simulink model "boggieDynamics_2021"  (Simulink 10.3)
settings: Solver=VariableStepAuto  StartTime=0.0  StopTime=10.0  RelTol=1e-3
undefined symbols (not defined in the file or in its folder): cg_suelo, g, m, x_guid12, x_guid34, x_lev12, x_lev34, y_lev13, y_lev24, z_guid, z_lev, z_lim
libraries: shared6dof x1
settings Model: Creator=aceao  LastModifiedBy=aceao
settings SolverCC: AlgebraicLoopSolver=Auto
settings DataIOCC: SaveFormat=Dataset  SignalLoggingSaveFormat=Dataset  ReturnWorkspaceOutputs=on
settings OptimizationCC: BlockReduction=off  BooleanDataType=off  ExpressionDepthLimit=128  LifeSpan=auto
settings DebuggingCC: SaveWithParameterizedLinksMsg=none  UnderspecifiedInitializationDetection=Simplified  SignalResolutionControl=TryResolveAllWithWarning  FcnCallInpInsideContextMsg=error  UnconnectedInputMsg=none  UnconnectedOutputMsg=none  UnconnectedLineMsg=none  StateNameClashWarn=none  SFUnexpectedBacktrackingDiag=error  SFNoUnconditionalDefaultTransitionDiag=error  SFExecutionAtInitializationDiag=warning  SFMachineParentedDataDiag=error  ArithmeticOperatorsInVariantConditions=error
settings HardwareCC: ProdBitPerPointer=64  ProdBitPerSizeT=64  ProdBitPerPtrDiffT=64  ProdLargestAtomicFloat=Float  ProdIntDivRoundTo=Zero  ProdEndianess=LittleEndian  ProdWordSize=64  ProdHWDeviceType=Intel->x86-64 (Windows64)  TargetUnknown=on
settings ModelReferenceCC: EnableRefExpFcnMdlSchedulingChecks=off
settings SFSimCC: SimUseLocalCustomCode=on  CustomCodeUndefinedFunction=FilterOut
settings RTWCC: RTWUseLocalCustomCode=on  DLArmComputeVersion=20.02.1
settings CodeAppCC: StateflowObjectComments=off
settings GRTTargetCC: TargetLangStandard=C99 (ISO)  CombineOutputUpdateFcns=on  GRTInterface=off
settings ConfigComp: CovMetricSettings=dwe  CovSaveCumulativeToWorkspaceVar=off  CovSaveSingleToWorkspaceVar=off  CovExternalEMLEnable=on

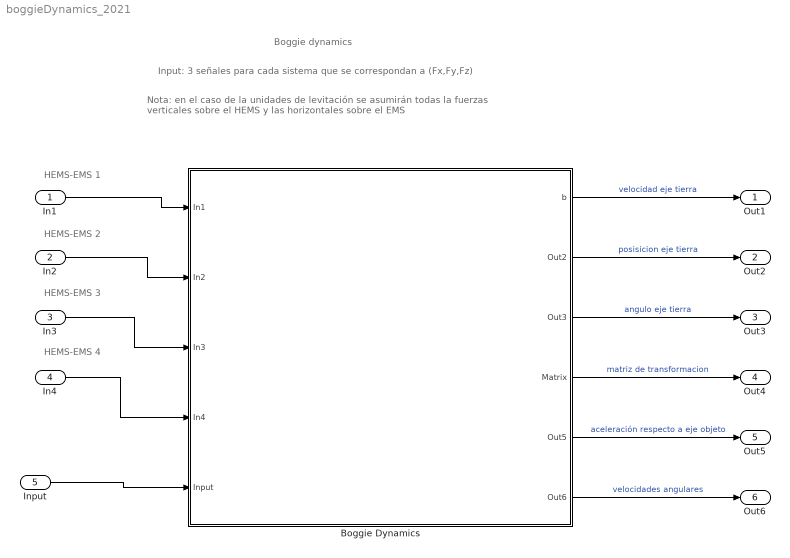
== system boggieDynamics_2021 ==
  note: Input: 3 señales para cada sistema que se correspondan a (Fx,Fy,Fz)
  note: Boggie dynamics
  note: HEMS-EMS 3
  note: HEMS-EMS 1
  note: HEMS-EMS 4
  note: HEMS-EMS 2
  note: Nota: en el caso de la unidades de levitación se asumirán todas la fuerzas
      | verticales sobre el HEMS y las horizontales sobre el EMS
  In1 : Inport
  In2 : Inport  Port=2
  In3 : Inport  Port=3
  In4 : Inport  Port=4
  Input : Inport  Port=5
  Boggie Dynamics : Subsystem
      mask Display: image('C:\UPV\Hyperloop\Levitacion\ejes.png'); % Use "Edit Image" on toolstrip to change.
  Out1 : Outport
  Out2 : Outport  Port=2
  Out3 : Outport  Port=3
  Out4 : Outport  Port=4
  Out5 : Outport  Port=5
  Out6 : Outport  Port=6
  wires:
  Boggie Dynamics/2(Out2) -> Out2/1  "posisicion eje tierra"
  Boggie Dynamics/3(Out3) -> Out3/1  "angulo eje tierra"
  Boggie Dynamics/1(b) -> Out1/1  "velocidad eje tierra"
  In1/1 -> Boggie Dynamics/1(In1)
  In2/1 -> Boggie Dynamics/2(In2)
  In3/1 -> Boggie Dynamics/3(In3)
  In4/1 -> Boggie Dynamics/4(In4)
  Boggie Dynamics/6(Out6) -> Out6/1  "velocidades angulares"
  Boggie Dynamics/5(Out5) -> Out5/1  "aceleración respecto a eje objeto"
  Boggie Dynamics/4(Matrix) -> Out4/1  "matriz de transformacion"
  Input/1 -> Boggie Dynamics/5(Input)

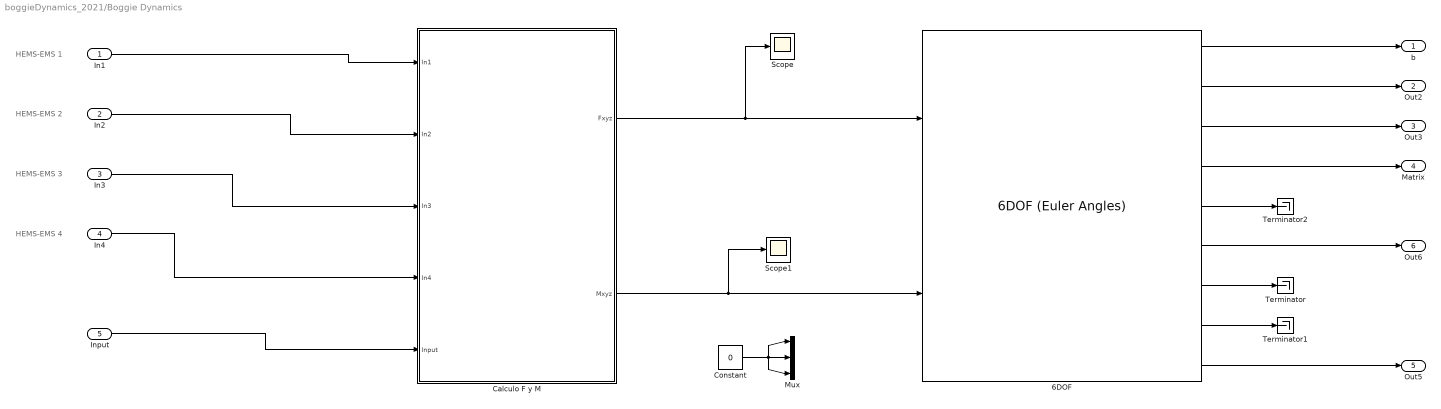
== system boggieDynamics_2021/Boggie Dynamics ==
  note: HEMS-EMS 1
  note: HEMS-EMS 2
  note: HEMS-EMS 3
  note: HEMS-EMS 4
  In1 : Inport
  In2 : Inport  Port=2
  In3 : Inport  Port=3
  In4 : Inport  Port=4
  Input : Inport  Port=5
  "6DOF " : shared6dof/6DOF (Euler Angles)  units=Metric (MKS)  mtype=Fixed  rep=Euler Angles  xme_0=[0 0.001 cg_suelo]  Vm_0=[0 0 0]  eul_0=[0 0 0]  pm_0=[0 0 0]  mass_0=m  mass_e=0.5  mass_f=2.0  inertia=I  inertia_e=eye(3)  inertia_f=2*eye(3)  k_quat=1.0  vre_flag=on  abi_flag=on  aMode=0  xme_statename=''  Vm_statename=''  eul_statename=''  quat_statename=''  pm_statename=''  mass_statename=''
  Calculo F y M : Subsystem
  Constant : Constant  Value=0
  Mux : Mux  Inputs=3
  Scope : Scope
  Scope1 : Scope
  Terminator : Terminator
  Terminator1 : Terminator
  Terminator2 : Terminator
  b : Outport
  Out2 : Outport  Port=2
  Out3 : Outport  Port=3
  Matrix : Outport  Port=4
  Out5 : Outport  Port=5
  Out6 : Outport  Port=6
  wires:
  "6DOF "/1 -> b/1
  "6DOF "/2 -> Out2/1
  "6DOF "/3 -> Out3/1
  In1/1 -> Calculo F y M/1(In1)
  In2/1 -> Calculo F y M/2(In2)
  In3/1 -> Calculo F y M/3(In3)
  In4/1 -> Calculo F y M/4(In4)
  "6DOF "/6 -> Out6/1
  "6DOF "/8 -> Terminator1/1
  "6DOF "/7 -> Terminator/1
  Calculo F y M/1(Fxyz) -> Scope/1, "6DOF "/1
  "6DOF "/4 -> Matrix/1
  "6DOF "/9 -> Out5/1
  "6DOF "/5 -> Terminator2/1
  Constant/1 -> Mux/3, Mux/1, Mux/2
  Input/1 -> Calculo F y M/5(Input)
  Calculo F y M/2(Mxyz) -> Scope1/1, "6DOF "/2

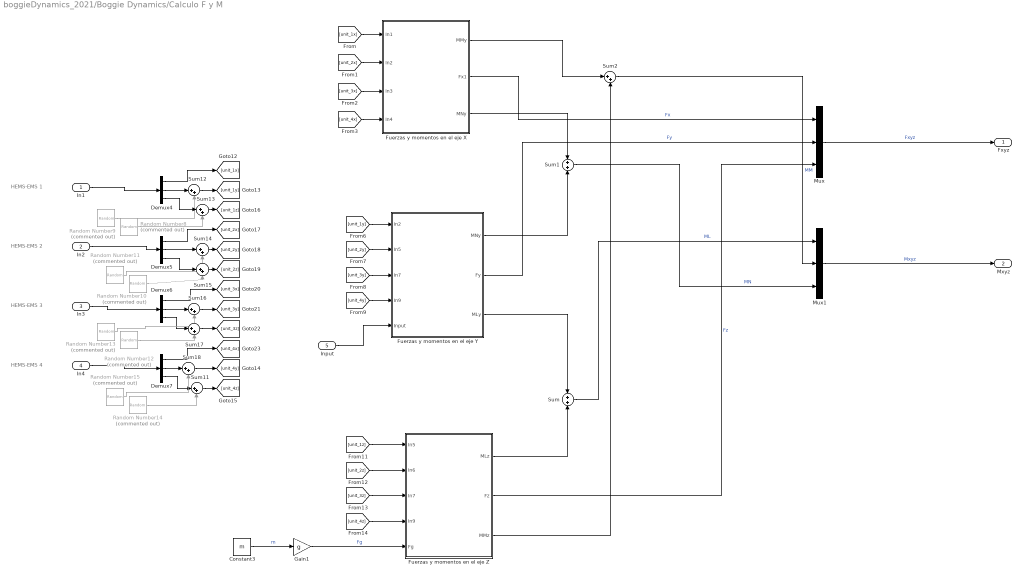
== system boggieDynamics_2021/Boggie Dynamics/Calculo F y M ==
  note: HEMS-EMS 3
  note: HEMS-EMS 1
  note: HEMS-EMS 4
  note: HEMS-EMS 2
  In1 : Inport
  In2 : Inport  Port=2
  In3 : Inport  Port=3
  In4 : Inport  Port=4
  Input : Inport  Port=5
  Constant3 : Constant  Value=m
  Demux{4..7} (4 alike) : Demux  Outputs=3
  Fuerzas y momentos en el eje X : Subsystem
  Fuerzas y momentos en el eje Y : Subsystem
  Fuerzas y momentos en el eje Z : Subsystem
  Gain1 : Gain  Gain=g
  Mux : Mux  Inputs=3
  Mux1 : Mux  Inputs=3
  Random Number10 : RandomNumber  Commented=on  Variance=20  Seed=3  SampleTime=0.1
  Random Number11 : RandomNumber  Commented=on  Variance=20  Seed=2  SampleTime=0.1
  Random Number12 : RandomNumber  Commented=on  Variance=20  Seed=5  SampleTime=0.1
  Random Number13 : RandomNumber  Commented=on  Variance=20  Seed=4  SampleTime=0.1
  Random Number14 : RandomNumber  Commented=on  Variance=20  Seed=7  SampleTime=0.1
  Random Number15 : RandomNumber  Commented=on  Variance=20  Seed=6  SampleTime=0.1
  Random Number8 : RandomNumber  Commented=on  Variance=20  Seed=1  SampleTime=0.1
  Random Number9 : RandomNumber  Commented=on  Variance=20  SampleTime=0.1
  Sum : Sum
  Sum1 : Sum
  Sum{2,11..18} (9 alike) : Sum  Inputs=|++
  Fxyz : Outport
  Mxyz : Outport  Port=2
  wires:
  Constant3/1 -> Gain1/1  "m"
  Sum2/1 -> Mux1/2  "MM"
  Mux/1 -> Fxyz/1  "Fxyz"
  Mux1/1 -> Mxyz/1  "Mxyz"
  Sum1/1 -> Mux1/3  "MN"
  Sum/1 -> Mux1/1  "ML"
  Fuerzas y momentos en el eje Y/2(Fy) -> Mux/2  "Fy"
  Fuerzas y momentos en el eje Y/1(MNy) -> Sum1/2
  Gain1/1 -> Fuerzas y momentos en el eje Z/5(Fg)  "Fg"
  Fuerzas y momentos en el eje Z/2(Fz) -> Mux/3  "Fz"
  Fuerzas y momentos en el eje Z/1(MLz) -> Sum/2
  [unit_4y] -> Fuerzas y momentos en el eje Y/4(In9)
  [unit_1y] -> Fuerzas y momentos en el eje Y/1(In2)
  [unit_2y] -> Fuerzas y momentos en el eje Y/2(In5)
  [unit_3y] -> Fuerzas y momentos en el eje Y/3(In7)
  [unit_1z] -> Fuerzas y momentos en el eje Z/1(In5)
  [unit_3z] -> Fuerzas y momentos en el eje Z/3(In7)
  [unit_2z] -> Fuerzas y momentos en el eje Z/2(In6)
  [unit_4z] -> Fuerzas y momentos en el eje Z/4(In9)
  Fuerzas y momentos en el eje Z/3(MMz) -> Sum2/2
  Fuerzas y momentos en el eje Y/3(MLy) -> Sum/1
  [unit_2x] -> Fuerzas y momentos en el eje X/2(In2)
  [unit_1x] -> Fuerzas y momentos en el eje X/1(In1)
  [unit_3x] -> Fuerzas y momentos en el eje X/3(In3)
  [unit_4x] -> Fuerzas y momentos en el eje X/4(In4)
  Fuerzas y momentos en el eje X/3(MNy) -> Sum1/1
  Fuerzas y momentos en el eje X/2(Fx1) -> Mux/1  "Fx"
  Fuerzas y momentos en el eje X/1(MMy) -> Sum2/1
  Input/1 -> Fuerzas y momentos en el eje Y/5(Input)
  Random Number9/1 -> Sum12/2
  Sum17/1 -> [unit_3z]
  Sum18/1 -> [unit_4y]
  Sum15/1 -> [unit_2z]
  Sum14/1 -> [unit_2y]
  Sum11/1 -> [unit_4z]
  Sum16/1 -> [unit_3y]
  Demux5/1 -> [unit_2x]
  Sum13/1 -> [unit_1z]
  Demux4/1 -> [unit_1x]
  Demux7/2 -> Sum18/1
  In1/1 -> Demux4/1
  Demux5/3 -> Sum15/1
  Demux6/2 -> Sum16/1
  Demux7/1 -> [unit_4x]
  Demux5/2 -> Sum14/1
  In4/1 -> Demux7/1
  In2/1 -> Demux5/1
  Sum12/1 -> [unit_1y]
  Demux7/3 -> Sum11/1
  Demux6/3 -> Sum17/1
  Random Number11/1 -> Sum14/2
  Random Number8/1 -> Sum13/2
  Demux4/2 -> Sum12/1
  Random Number15/1 -> Sum18/2
  Demux4/3 -> Sum13/1
  Demux6/1 -> [unit_3x]
  Random Number13/1 -> Sum16/2
  Random Number14/1 -> Sum11/2
  In3/1 -> Demux6/1
  Random Number10/1 -> Sum15/2
  Random Number12/1 -> Sum17/2

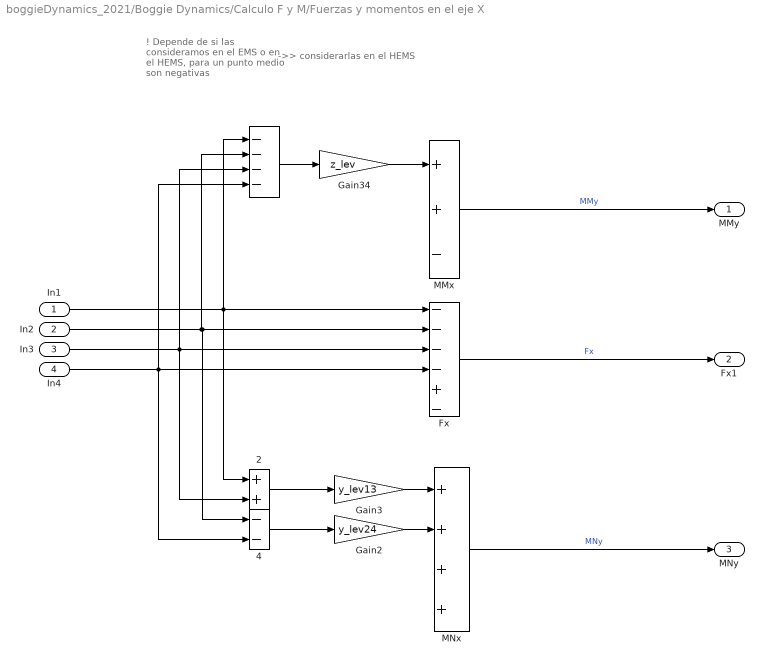
== system boggieDynamics_2021/Boggie Dynamics/Calculo F y M/Fuerzas y momentos en el eje X ==
  note: ! Depende de si las consideramos en el EMS o en el HEMS,
      | para un punto medio son negativas
  note: ->> considerarlas en el HEMS
  In1 : Inport
  In2 : Inport  Port=2
  In3 : Inport  Port=3
  In4 : Inport  Port=4
  " " : Sum  Inputs=----
  " 2" : Sum
  " 4" : Sum  Inputs=--
  Fx : Sum  Inputs=----+-
  Gain2 : Gain  Gain=y_lev24
  Gain3 : Gain  Gain=y_lev13
  Gain34 : Gain  Gain=z_lev
  MMx : Sum  Inputs=++-
  MNx : Sum  Inputs=++++
  MMy : Outport
  Fx1 : Outport  Port=2
  MNy : Outport  Port=3
  wires:
  In1/1 -> " 2"/1, " "/1, Fx/1
  In2/1 -> " "/2, " 4"/1, Fx/2
  Fx/1 -> Fx1/1  "Fx"
  MMx/1 -> MMy/1  "MMy"
  In4/1 -> " 4"/2, " "/4, Fx/4
  In3/1 -> " "/3, " 2"/2, Fx/3
  Gain34/1 -> MMx/1
  MNx/1 -> MNy/1  "MNy"
  " "/1 -> Gain34/1
  " 4"/1 -> Gain2/1
  " 2"/1 -> Gain3/1
  Gain3/1 -> MNx/1
  Gain2/1 -> MNx/2

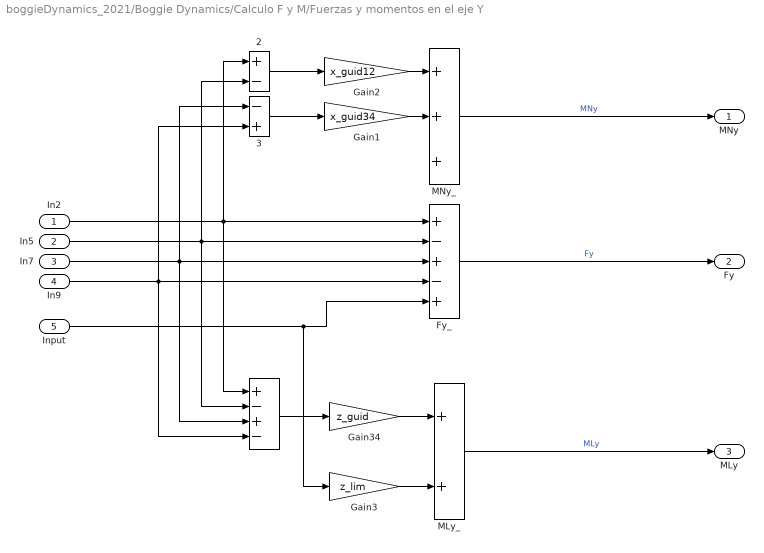
== system boggieDynamics_2021/Boggie Dynamics/Calculo F y M/Fuerzas y momentos en el eje Y ==
  In2 : Inport
  In5 : Inport  Port=2
  In7 : Inport  Port=3
  In9 : Inport  Port=4
  Input : Inport  Port=5
  " " : Sum  Inputs=+-+-
  " 2" : Sum  Inputs=+-
  " 3" : Sum  Inputs=-+
  Fy_ : Sum  Inputs=+-+-+
  Gain1 : Gain  Gain=x_guid34
  Gain2 : Gain  Gain=x_guid12
  Gain3 : Gain  Gain=z_lim
  Gain34 : Gain  Gain=z_guid
  MLy_ : Sum
  MNy_ : Sum  Inputs=+++
  MNy : Outport
  Fy : Outport  Port=2
  MLy : Outport  Port=3
  wires:
  Fy_/1 -> Fy/1  "Fy"
  MLy_/1 -> MLy/1  "MLy"
  In7/1 -> Fy_/3, " "/3, " 3"/1
  In9/1 -> " "/4, " 3"/2, Fy_/4
  In2/1 -> " "/1, " 2"/1, Fy_/1
  In5/1 -> " "/2, Fy_/2, " 2"/2
  MNy_/1 -> MNy/1  "MNy"
  " 3"/1 -> Gain1/1
  " 2"/1 -> Gain2/1
  Gain1/1 -> MNy_/2
  Gain2/1 -> MNy_/1
  " "/1 -> Gain34/1
  Gain34/1 -> MLy_/1
  Input/1 -> Gain3/1, Fy_/5
  Gain3/1 -> MLy_/2

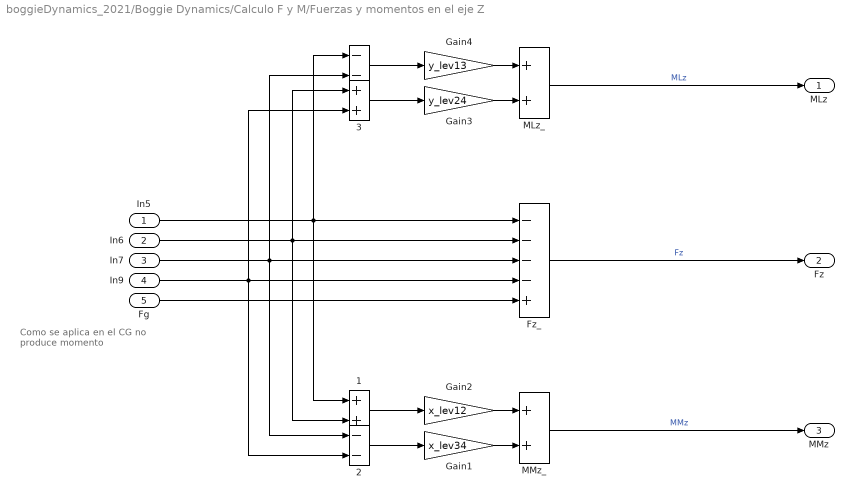
== system boggieDynamics_2021/Boggie Dynamics/Calculo F y M/Fuerzas y momentos en el eje Z ==
  note: Como se aplica en el CG
      |  no produce momento
  In5 : Inport
  In6 : Inport  Port=2
  In7 : Inport  Port=3
  In9 : Inport  Port=4
  Fg : Inport  Port=5
  " " : Sum  Inputs=--
  " 1" : Sum
  " 2" : Sum  Inputs=--
  " 3" : Sum
  " MLz_" : Sum
  " MMz_" : Sum
  Fz_ : Sum  Inputs=----+
  Gain1 : Gain  Gain=x_lev34
  Gain2 : Gain  Gain=x_lev12
  Gain3 : Gain  Gain=y_lev24
  Gain4 : Gain  Gain=y_lev13
  MLz : Outport
  Fz : Outport  Port=2
  MMz : Outport  Port=3
  wires:
  In6/1 -> " 1"/2, Fz_/2, " 3"/1
  " MLz_"/1 -> MLz/1  "MLz"
  Fg/1 -> Fz_/5
  In9/1 -> Fz_/4, " 2"/2, " 3"/2
  In5/1 -> " 1"/1, " "/1, Fz_/1
  In7/1 -> " 2"/1, Fz_/3, " "/2
  Fz_/1 -> Fz/1  "Fz"
  " MMz_"/1 -> MMz/1  "MMz"
  " 3"/1 -> Gain3/1
  " "/1 -> Gain4/1
  Gain4/1 -> " MLz_"/1
  Gain3/1 -> " MLz_"/2
  Gain2/1 -> " MMz_"/1
  " 2"/1 -> Gain1/1
  Gain1/1 -> " MMz_"/2
  " 1"/1 -> Gain2/1
